simulink model "RS232_HFC_loopback_1P"  (Simulink 7.8)
settings: Solver=VariableStepDiscrete  StartTime=0.0  StopTime=Inf  FixedStep=Ts/4  RelTol=1e-3
PreLoadFcn:
  | clear all;
  | close all;
  | clc;
  | 
  | Ts = 1;          % clk (period)
StartFcn:
  | clc;
  | close all;
  | 
  | %
  | %   RS232 port initialization
  | %
  | PORTNAME = 'COM34';
  | fprintf('\nOpening RS232 port %s ...... ', PORTNAME);
  | s1 = serial(PORTNAME,'BaudRate',9600,'Parity','none','DataBits',8);
  | set(s1, 'FlowControl', 'none');
  | set(s1, 'InputBufferSize', 64);
  | set(s1, 'OutputBufferSize', 1);
  | fopen(s1);
  | s1.RecordDetail = 'verbose';
  | s1.RecordName = 'lb.txt';
  | record(s1,'on')
  | fprintf('\nRS232 port %s activated\n', PORTNAME);
  | 
  | b2o_s1 = uint8(0);
  | d2o_s1 = uint8(0);
  | b2r_s1 = uint8(0);
  | d2r_s1 = uint8(0);
  | rts_s1 = uint8(0);
  | cts_s1 = uint8(0);
StopFcn:
  | %
  | %   RS232 ports release
  | %
  | disp(' ');
  | disp('Deactivating RS232 port ......');
  | 
  | fclose(s1)
  | delete(s1)
  | clear s1
  | 
  | fprintf('RS232 port %s deactivated\n', PORTNAME);
libraries: simulink x2
settings Model: Creator=theodore  LastModifiedBy=theodore
settings DebuggingCC: SolverPrmCheckMsg=none
settings CodeAppCC: CustomSymbolStrType=$N$R$M_T

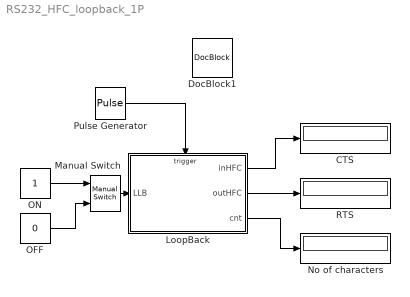
== system RS232_HFC_loopback_1P ==
  CTS : Display
  DocBlock1 : simulink/Model-Wide Utilities/DocBlock  DocumentType=Text
  LoopBack : Stateflow chart  TreatAsAtomicUnit=on
  Manual Switch : simulink/Signal Routing/Manual Switch  sw=1  action=0  varsize=off
  No of characters : Display
  OFF : Constant  Value=0
  ON : Constant
  Pulse Generator : DiscretePulseGenerator  PulseType=Time based  Period=Ts  PulseWidth=50
  RTS : Display
  wires:
  LoopBack/3(cnt) -> No of characters/1
  LoopBack/2(outHFC) -> RTS/1
  LoopBack/1(inHFC) -> CTS/1
  Pulse Generator/1 -> LoopBack/Trigger
  Manual Switch/1 -> LoopBack/1(LLB)
  ON/1 -> Manual Switch/1
  OFF/1 -> Manual Switch/2

== stateflow chart LoopBack ==
  state HFC [parallel]
    settings: executionOrder=1
    state HFCcon
      ml('CTS_1');
      LBstatus = ml.cts_s1;
      inHFC = LBstatus;
      LBstatus = LBstatus & LLB;
      ml.rts_s1 = LBstatus;
      outHFC = LBstatus;
      ml('RTS_1');
    (default) -> HFCcon
    HFCcon -> HFCcon
  state TxR [parallel]
    settings: executionOrder=2
    state RxState
      en: ml('DIn_1');
      Val = ml.d2r_s1;
      cnt = cnt + 1;
    state IniState
    state TxState
      en: ml.d2o_s1 = Val;
      ml('DOut_1');
    (default) -> IniState : {cnt = 0;}
    (junction 9) -> IniState [order 1] : [LBstatus == 0  || ml.b2o_s1 > 0 ||  ml.b2r_s1 == 0 ]
    TxState -> IniState
    IniState -> (junction 9) : {ml('B2O_1'); ml('B2R_1'); }
    (junction 9) -> RxState [order 2]
    RxState -> TxState : [LBstatus == 1 ]
  data: inHFC output double; outHFC output double; Val local double; cnt output double; LBstatus local double =0; LLB input double
  events: CLK input RISING_EDGE_EVENT
